simulink model "Differential_Drive_Robot_Dynamics_Model"  (R2017b)
settings: Solver=VariableStepAuto  StartTime=0.0  StopTime=10  RelTol=1e-3
settings Model: Creator=Jesus  LastModifiedBy=Jesus

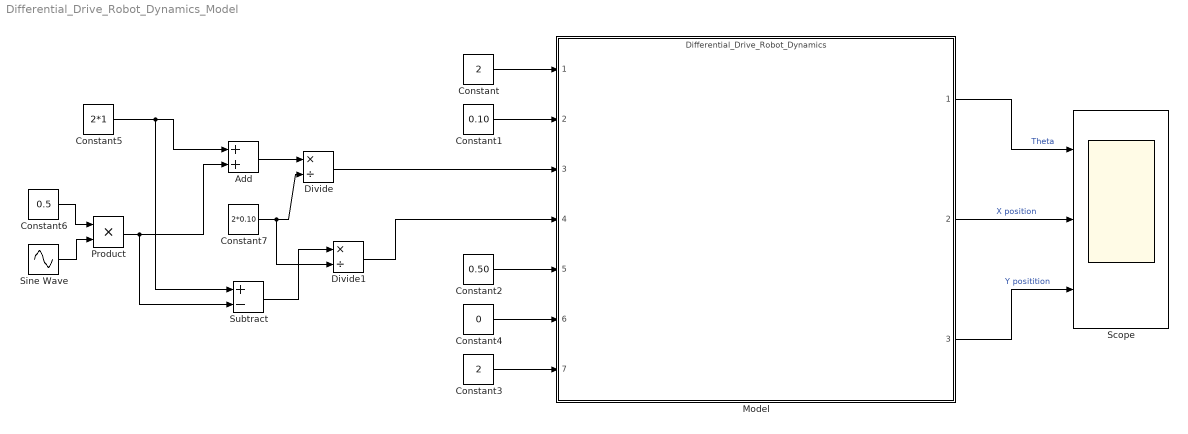
== system Differential_Drive_Robot_Dynamics_Model ==
  Add : Sum
  Constant : Constant  Value=2
  Constant1 : Constant  Value=0.10
  Constant2 : Constant  Value=0.50
  Constant3 : Constant  Value=2
  Constant4 : Constant  Value=0
  Constant5 : Constant  Value=2*1
  Constant6 : Constant  Value=0.5
  Constant7 : Constant  Value=2*0.10
  Divide : Product  Inputs=*/
  Divide1 : Product  Inputs=*/
  Model : ModelReference  ModelNameDialog=Differential_Drive_Robot_Dynamics.slx  SimulationMode=Normal  ModelReferenceVersion=1.3
  Product : Product
  Scope : Scope  NumInputPorts=3
  Sine Wave : Sin  Frequency=100  SampleTime=0
  Subtract : Sum  Inputs=+-
  wires:
  Constant/1 -> Model/1
  Constant1/1 -> Model/2
  Constant2/1 -> Model/5
  Constant3/1 -> Model/7
  Model/1 -> Scope/1  "Theta"
  Model/2 -> Scope/2  "X position"
  Model/3 -> Scope/3  "Y positition"
  Constant4/1 -> Model/6
  Constant5/1 -> Add/1, Subtract/1
  Sine Wave/1 -> Product/2
  Constant6/1 -> Product/1
  Product/1 -> Subtract/2, Add/2
  Add/1 -> Divide/1
  Constant7/1 -> Divide1/2, Divide/2
  Divide/1 -> Model/3
  Subtract/1 -> Divide1/1
  Divide1/1 -> Model/4
